simulink model "em"  (R2023b)
settings: Solver=FixedStepDiscrete  StartTime=0.0  StopTime=3180  FixedStep=0.015  RelTol=1e-3
settings Model: TunableVars=FINISHED_SMOOTHENING_IC,LAST_TVS_PERMIT_IC,w,V,k_min,dk,dk_thresh,alpha,k_IC  TunableVarsStorageClass=Auto,Auto,Auto,Auto,Auto,Auto,Auto,Auto,Auto  TunableVarsTypeQualifier=,,,,,,,,  Creator=Inver  LastModifiedBy=Inver
settings DataIOCC: ExternalInput=ds_em_test_v0.getElement('rTVS'),ds_em_test_v0.getElement('rEQUAL'),ds_em_test_v0.getElement('V'),ds_em_test_v0.getElement('w'),ds_em_test_v0.getElement('TVS_STATE')  LoadExternalInput=on
settings OptimizationCC: DefaultParameterBehavior=Inlined  GainParamInheritBuiltInType=on  UseFloatMulNetSlope=on  UseSpecifiedMinMax=on  InlineInvariantSignals=on  StrengthReduction=on  PassReuseOutputArgsAs=Individual arguments  ZeroExternalMemoryAtStartup=off  ZeroInternalMemoryAtStartup=off  NoFixptDivByZeroProtection=on  EfficientFloat2IntCast=on  LifeSpan=1  OptimizeBlockOrder=speed  DifferentSizesBufferReuse=on  OptimizationPriority=Speed  MultiThreadedLoops=on  EfficientTunableParamExpr=on
settings DebuggingCC: ReadBeforeWriteMsg=DisableAll  WriteAfterWriteMsg=DisableAll  WriteAfterReadMsg=DisableAll  MultiTaskDSMMsg=none  ParameterTunabilityLossMsg=error
settings HardwareCC: ProdBitPerPointer=32  ProdBitPerSizeT=32  ProdBitPerPtrDiffT=32  ProdLargestAtomicInteger=Long  ProdLargestAtomicFloat=Double  ProdWordSize=32  ProdLongLongMode=on  ProdHWDeviceType=ARM Compatible->ARM Cortex-M
settings ModelReferenceCC: UpdateModelReferenceTargets=IfOutOfDate
settings SFSimCC: SFSimEcho=off  MATLABDynamicMemAlloc=off
settings RTWCC: Description=Embedded Coder  SystemTargetFile=ert.tlc  GenCodeOnly=on  PackageGeneratedCodeAndArtifacts=on  TemplateMakefile=ert_default_tmf  Toolchain=GNU Tools for ARM Embedded Processors  BuildConfiguration=Faster Runs
settings CodeAppCC: ForceParamTrailComments=on  IgnoreCustomStorageClasses=off  SimulinkDataObjDesc=on  CustomSymbolStrGlobalVar=rt$N$M_em  CustomSymbolStrType=$N$M_em  CustomSymbolStrBlkIO=$N$M  SimulinkBlockComments=off
settings ERTTargetCC: TargetLangStandard=C99 (ISO)  GenerateSampleERTMain=on  CombineSignalStateStructs=on  SuppressErrorStatus=on  CodeInterfacePackaging=Reusable function  SupportNonFinite=off  SupportComplex=off  InlinedParameterPlacement=NonHierarchical  RootIOFormat=Structure reference  ERTCustomFileTemplate=example_file_process.tlc  GlobalDataDefinition=InSeparateSourceFile  DataDefinitionFile=data.c  GlobalDataReference=InSeparateHeaderFile  ERTFilePackagingFormat=CompactWithDataFile  DataReferenceFile=data.h

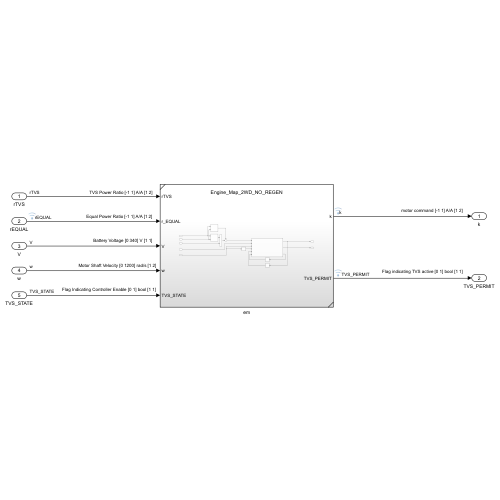
[thumbnail: Simulink's stored preview of the top-level diagram]
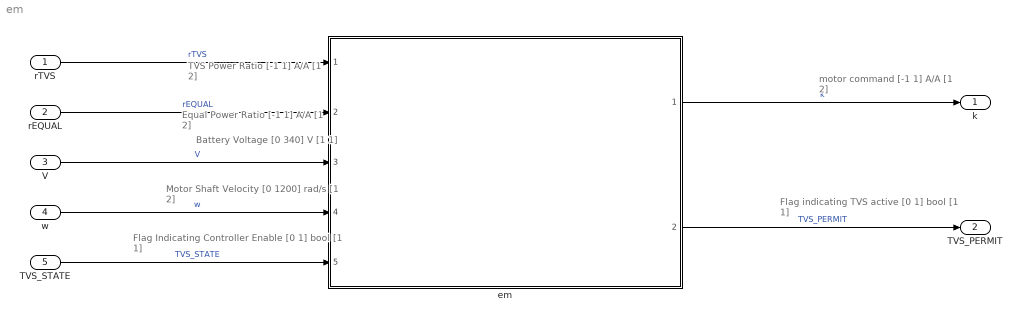
== system em ==
  note: motor command [-1 1] A/A [1 2]
  note: Flag indicating TVS active [0 1] bool [1 1]
  note: Motor Shaft Velocity [0 1200] rad/s [1 2]
  note: Equal Power Ratio [-1 1] A/A [1 2]
  note: Battery Voltage [0 340] V [1 1]
  note: TVS Power Ratio [-1 1] A/A [1 2]
  note: Flag Indicating Controller Enable [0 1] bool [1 1]
  rTVS : Inport  PortDimensions=[1 2]
  rEQUAL : Inport  Port=2  PortDimensions=[1 2]
  V : Inport  Port=3  PortDimensions=[1 1]
  w : Inport  Port=4  PortDimensions=[1 2]
  TVS_STATE : Inport  Port=5  PortDimensions=[1 1]
  em : Subsystem  ReferencedSubsystem=Engine_Map_2WD_NO_REGEN
  k : Outport
  TVS_PERMIT : Outport  Port=2
  wires:
  em/2 -> TVS_PERMIT/1  "TVS_PERMIT"
  em/1 -> k/1  "k"
  rEQUAL/1 -> em/2  "rEQUAL"
  rTVS/1 -> em/1  "rTVS"
  V/1 -> em/3  "V"
  w/1 -> em/4  "w"
  TVS_STATE/1 -> em/5  "TVS_STATE"
